simulink model "inverter"  (R2025a)
settings: Solver=FixedStepAuto  StartTime=0.0  StopTime=2  RelTol=1e-3
values from neighbouring files (symbols this model uses):
  Kd = 0    [optimizasyon_baslat.m]
libraries: spsSeriesRLCBranchLib x5, spsDiodeLib x4, spsMosfetLib x4, spsRMSLib x3, spsVoltageMeasurementLib x3, spsControlledVoltageSourceLib x1, spsCurrentMeasurementLib x1, slpidlib x1, eePwmGenerator x1, simulink x1, spsBreakerLib x1, sps_lib x1
settings Model: Creator=TOPALOĞLU  LastModifiedBy=TOPALOĞLU

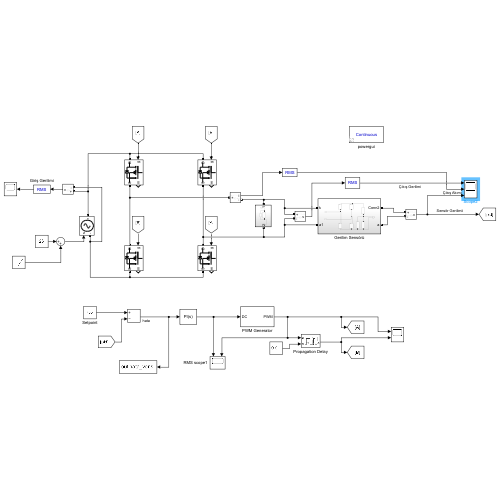
[thumbnail: Simulink's stored preview of the top-level diagram]
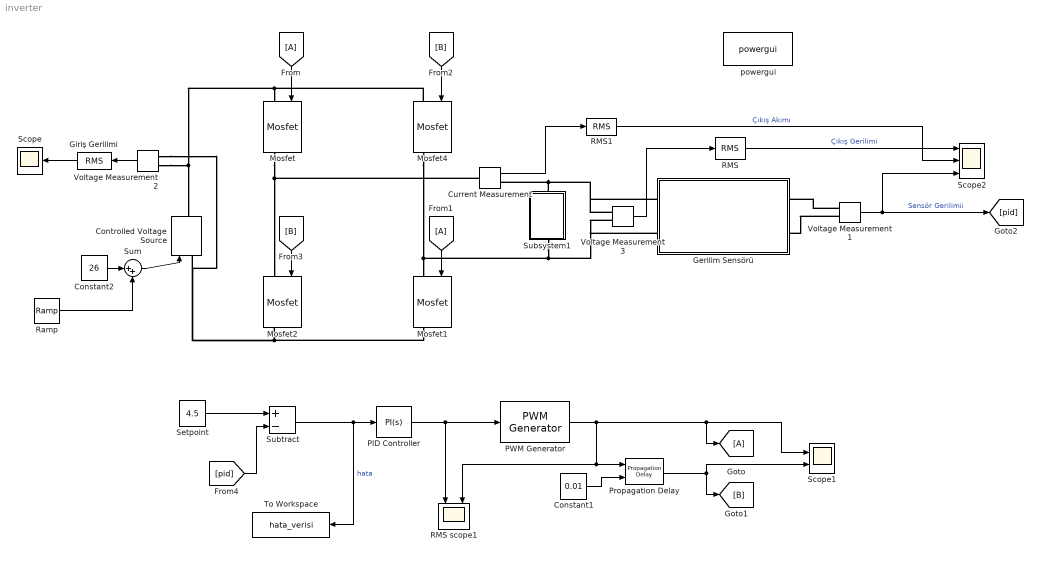
== system inverter ==
  Constant1 : Constant  Value=0.01
  Constant2 : Constant  Value=26
  Controlled Voltage Source : spsControlledVoltageSourceLib/Controlled Voltage Source  Initialize=on  Source_Type=DC  Amplitude=0  Phase=0  Frequency=0  Measurements=None
  Current Measurement : spsCurrentMeasurementLib/Current Measurement  PhasorSimulation=off  OutputType=Complex  PSBequivalent=0
  From : From
  From1 : From
  Gerilim Sensörü : Subsystem
  Giriş Gerilimi : spsRMSLib/RMS  TrueRMS=on  Freq=50  RMSInit=26  Ts=0
  Goto : Goto
  Mosfet{,1..2,4} (4 alike) : spsMosfetLib/Mosfet  Ron=0.1  Lon=0  Rd=0.01  Vfd=0  IC=0  Rs=inf  Cs=0  Measurements=on
  PID Controller : slpidlib/PID Controller  Controller=PI  Form=Parallel  TimeDomain=Continuous-time  UseExternalTs=off  SampleTime=-1  IntegratorMethod=Forward Euler  FilterMethod=Forward Euler  ControllerParametersSource=internal  P=0.059307  I=1.9095  UseKiTs=off  D=Kd  UseExternalDerivativeSource=off  N=100  UseFilter=on  TunerSelectOption=Transfer Function Based (PID Tuner App)  InitialConditionSource=internal  InitialConditionForIntegrator=0  InitialConditionForFilter=0  DifferentiatorICPrevScaledInput=0  ExternalReset=none  TrackingMode=off  Kt=1  LimitOutput=off  SatLimitsSource=internal  UpperSaturationLimit=0.95  LowerSaturationLimit=0  LinearizeAsGain=on  AntiWindupMode=clamping  Kb=1  LimitIntegrator=off  UpperIntegratorSaturationLimit=inf  LowerIntegratorSaturationLimit=-inf  POutMin=[]  POutMax=[]  IOutMin=[]  IOutMax=[]  DOutMin=[]  DOutMax=[]  NOutMin=[]  NOutMax=[]  SumOutMin=[]  SumOutMax=[]  SaturationOutMin=[]  SaturationOutMax=[]  PParamMin=[]  PParamMax=[]  IParamMin=[]  IParamMax=[]  DParamMin=[]  DParamMax=[]  NParamMin=[]  NParamMax=[]  KbParamMin=[]  KbParamMax=[]  KtParamMin=[]  KtParamMax=[]  KbOutMin=[]  KbOutMax=[]  KtOutMin=[]  KtOutMax=[]  IntegratorOutMin=[]  IntegratorOutMax=[]  FilterOutMin=[]  FilterOutMax=[]  SumI1OutMin=[]  SumI1OutMax=[]  SumI2OutMin=[]  SumI2OutMax=[]  SumI3OutMin=[]  SumI3OutMax=[]  SumI4OutMin=[]  SumI4OutMax=[]  SumDOutMin=[]  SumDOutMax=[]  DifferentiatorOutMin=[]  DifferentiatorOutMax=[]  FilterDiffOutCoefMin=[]  FilterDiffOutCoefMax=[]  ReciprocalOutMin=[]  ReciprocalOutMax=[]  SumDenOutMin=[]  SumDenOutMax=[]  SumNumOutMin=[]  SumNumOutMax=[]  DivideOutMin=[]  DivideOutMax=[]  UdiffTsProdOutMin=[]  UdiffTsProdOutMax=[]  NTsProdOutMin=[]  NTsProdOutMax=[]  UintegralTsProdOutMin=[]  UintegralTsProdOutMax=[]  UngainTsProdOutMin=[]  UngainTsProdOutMax=[]  ClampingZeroOutDataTypeStr=Inherit: Inherit via back propagation  ClampingZeroOutMin=[]  ClampingZeroOutMax=[]  FilterDenConstantOutDataTypeStr=Inherit: Inherit via back propagation  FilterDenConstantOutMin=[]  FilterDenConstantOutMax=[]  PCopyOutDataTypeStr=Inherit: Inherit via back propagation  PCopyOutMin=[]  PCopyOutMax=[]  NCopyOutDataTypeStr=Inherit: Inherit via back propagation  NCopyOutMin=[]  NCopyOutMax=[]  IntegratorContinuousStateAttributes=''  IntegratorStateMustResolveToSignalObject=off  IntegratorRTWStateStorageClass=Auto  FilterContinuousStateAttributes=''  FilterStateMustResolveToSignalObject=off  FilterRTWStateStorageClass=Auto  ParallelPVariant=InternalParameters  IdealPVariant=Disabled  IVariant=InternalParameters  DVariant=Disabled  IntegratorVariant=Continuous  SatVariant=Disabled  AWVariant=Passthrough  PCopyVariant=Disabled  TRVariant=Disabled  FdbkBlocksVariant=Forward  IdealPFdbkVariant=Disabled  SatFdbkVariant=Disabled  DerivativeFilterVariant=Disabled  NVariant=Disabled  NCopyVariant=Disabled_SignalSpec  FilterICVariant=Disabled  IntegratorICVariant=InternalICs  ExternalResetVariant=Disabled  TRSumVariant=Passthrough  SumFdbkVariant=Disabled  SumVariant=Sum_PI  TsampFilterVariant=InternalTs  TsampNgainVariant=Passthrough  TsampIntegralVariant=Disabled_SignalSpec  ExternalSaturationOutDataTypeStr=Inherit: Same as second input  DerivativeSourceVariant=Disabled  PreIntVariant=InternalPreInt
  PWM Generator : eePwmGenerator/PWM Generator  CarrCount=Up  Tper=0.02  Tdelay=0  Ts=0
  Propagation Delay : PropagationDelay  RunAtFixedTimeIntervals=on  SampleTime=1e-5
  RMS : spsRMSLib/RMS  TrueRMS=on  Freq=50  RMSInit=12  Ts=0
  RMS scope1 : Scope  NumInputPorts=2
      settings: ActiveDisplayYMinimum=-0.11874999999999997  ActiveDisplayYMaximum=1.0687499999999999
  RMS1 : spsRMSLib/RMS  TrueRMS=on  Freq=50  RMSInit=12  Ts=0
  Ramp : simulink/Sources/Ramp  slope=-2  start=0.3  InitialOutput=0
  Scope : Scope
      settings: ActiveDisplayYMinimum=22.197503315644997  ActiveDisplayYMaximum=26.422499631625165  DataLoggingVariableName=ScopeData2
  Scope1 : Scope  NumInputPorts=2
      settings: SampleTime=5e-5  ActiveDisplayYMinimum=-1.5835891369267512  ActiveDisplayYMaximum=1.8370895793058766
  Scope2 : Scope  NumInputPorts=3
      settings: ActiveDisplayYMinimum=10.998473275040297  ActiveDisplayYMaximum=21.013740524637338  DataLoggingVariableName=ScopeData3
  Setpoint : Constant  Value=4.5
  Subsystem1 : Subsystem
      settings: PortSchema="{\"entries\":[{\"content\":{\"sides\":[{\"content\":{},\"type\":\"ConnectorPlacement.EquallySpacedRectSide\",\"uuid\":\"7486039e-ec59-494d-8c75-0b6bdb988410\"},{\"content\":{\"side\":\"RIGHT\"},\"type\":\"ConnectorPlacement.EquallySpacedRectSide\",\"uuid\":\"15f9885d-5be6-4b9d-bebb-8881537d42c9\"},{\"content\":{\"connectorIds\":[\"LConn1\"],\"side\":\"TOP\"},\"type\":\"ConnectorPlacement.EquallySpacedRectSide\",\"uuid\":\"8cabd63c-7798-48b1-8db3-4643120ccc1c\"},{\"content\":{\"connectorIds\":[\"RConn1\"],\"side\":\"BOTTOM\"},\"type\":\"ConnectorPlacement.EquallySpacedRectSide\",\"uuid\":\"bbf3fb16-ed9b-4739-ac92-1db30e999269\"}]},\"type\":\"ConnectorPlacement.EquallySpacedConnector\",\"uuid\":\"ea19a637-8e2a-4c18-aba2-8529bbc4d327\"}],\"packageUris\":[\"http://schema.mathworks.com/mf0/Connector/R2020b\"],\"version\":\"1.0\"}"
  Subtract : Sum  Inputs=+-
  Sum : Sum  Inputs=|++
  To Workspace : ToWorkspace  VariableName=hata_verisi  SampleTime=-1
      settings: Save2DSignal=2-D array (concatenate along first dimension)
  Voltage Measurement1 : spsVoltageMeasurementLib/Voltage Measurement  PhasorSimulation=off  OutputType=Complex  PSBequivalent=0
  Voltage Measurement2 : spsVoltageMeasurementLib/Voltage Measurement  PhasorSimulation=off  OutputType=Complex  PSBequivalent=0
  Voltage Measurement3 : spsVoltageMeasurementLib/Voltage Measurement  PhasorSimulation=off  OutputType=Complex  PSBequivalent=0
  powergui : sps_lib/powergui  Priority=1  SimulationMode=Continuous  SampleTime=5e-5  frequency=60  Iterations=50  frequencyindice=0  Pbase=100e6  ErrMax=1e-4  UnitsV=kV  UnitsW=MW  buscounter=0  FunctionMessages=off  echomessages=off  EnableUseOfTLC=off  CurrentSourceSwitches=off  DisableSnubberDevices=off  DisableRonSwitches=off  DisableVfSwitches=off  DisplayEquations=off  AutomaticDiscreteSolvers=off  SolverType=Tustin/Backward Euler (TBE)  Interpol=off  ExternalGateDelay=off  methode=off  Ts=100  x0status=blocks  SPID=on  SwTol=0  HookPort=off  NonlinearTolerance=1e-4  nMaxIteration=100  ContinueOnMaxIteration=off  RestoreLinks=warning  ResistiveCurrentMeasurement=off  Frange=[0:2:500]  Ylog=off  Xlog=on  ShowGrid=off  save=off  variable=ZData  structure=0  ZoomFFT=off  StartTime=0.0  cycles=1  DisplayStyle=1  fundamental=60  FreqAxis=off  MaxFrequency=1000  frequencyindicesteady=1  RmsSteady=1  display=off
  wires:
  [B] -> Mosfet4/1
  From1/1 -> Mosfet1/1
  Constant1/1 -> Propagation Delay/2
  Setpoint/1 -> Subtract/1
  Subtract/1 -> To Workspace/1, PID Controller/1  "hata"
  [B] -> Mosfet2/1
  PWM Generator/1 -> Propagation Delay/1, RMS scope1/2, Goto/1, Scope1/1
  From/1 -> Mosfet/1
  Propagation Delay/1 -> Scope1/2, [B]
  Constant2/1 -> Sum/1
  Ramp/1 -> Sum/2
  Sum/1 -> Controlled Voltage Source/1
  Giriş Gerilimi/1 -> Scope/1
  Voltage Measurement2/1 -> Giriş Gerilimi/1
  Voltage Measurement3/1 -> RMS/1
  RMS/1 -> Scope2/1  "Çıkış Gerilimi"
  Voltage Measurement1/1 -> [pid], Scope2/3  "Sensör Gerilimii"
  PID Controller/1 -> PWM Generator/1, RMS scope1/1
  Current Measurement/1 -> RMS1/1
  RMS1/1 -> Scope2/2  "Çıkış Akımı"
  [pid] -> Subtract/2
  connections:
  Mosfet4/LConn1 -- Voltage Measurement2/LConn1 -- Controlled Voltage Source/RConn1 -- Mosfet/LConn1
  Mosfet1/RConn1 -- Voltage Measurement2/LConn2 -- Controlled Voltage Source/LConn1 -- Mosfet2/RConn1
  Mosfet/RConn1 -- Current Measurement/LConn1 -- Mosfet2/LConn1
  Mosfet4/RConn1 -- Voltage Measurement3/LConn2 -- Gerilim Sensörü/LConn2 -- Subsystem1/RConn1 -- Mosfet1/LConn1
  Subsystem1/LConn1 -- Gerilim Sensörü/LConn1 -- Voltage Measurement3/LConn1 -- Current Measurement/RConn1
  Voltage Measurement1/LConn1 -- Gerilim Sensörü/RConn1
  Voltage Measurement1/LConn2 -- Gerilim Sensörü/RConn2

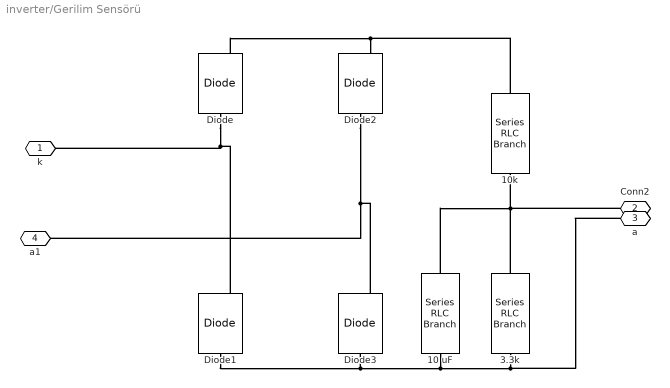
== system inverter/Gerilim Sensörü ==
  10 uF : spsSeriesRLCBranchLib/Series RLC Branch  LConnTagsString=__new0  RConnTagsString=__new0  BranchType=C  Resistance=1  Inductance=1e-3  SetiL0=off  InitialCurrent=0  Capacitance=10e-6  Setx0=off  InitialVoltage=0  Measurements=None
  10k : spsSeriesRLCBranchLib/Series RLC Branch  LConnTagsString=__new0  RConnTagsString=__new0  BranchType=R  Resistance=10000  Inductance=1e-3  SetiL0=off  InitialCurrent=0  Capacitance=10e-6  Setx0=off  InitialVoltage=0  Measurements=None
  3.3k : spsSeriesRLCBranchLib/Series RLC Branch  LConnTagsString=__new0  RConnTagsString=__new0  BranchType=R  Resistance=3300  Inductance=1e-3  SetiL0=off  InitialCurrent=0  Capacitance=10e-6  Setx0=off  InitialVoltage=0  Measurements=None
  Diode{,1..3} (4 alike) : spsDiodeLib/Diode  Ron=0.001  Lon=0  Vf=0.8  IC=0  UseSnubber=0  Rs=500  Cs=250e-9  Measurements=on
  k : PMIOPort  Side=Left
  Conn2 : PMIOPort  Port=2  Side=Right
  a : PMIOPort  Port=3  Side=Right
  a1 : PMIOPort  Port=4  Side=Left
  connections:
  Diode1/LConn1 -- 10 uF/RConn1 -- a/RConn1 -- 3.3k/RConn1 -- Diode3/LConn1
  Diode/LConn1 -- k/RConn1 -- Diode1/RConn1
  Diode3/RConn1 -- a1/RConn1 -- Diode2/LConn1
  3.3k/LConn1 -- Conn2/RConn1 -- 10 uF/LConn1 -- 10k/RConn1
  Diode/RConn1 -- 10k/LConn1 -- Diode2/RConn1

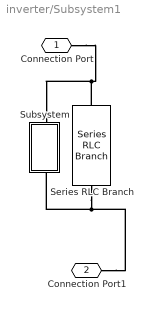
== system inverter/Subsystem1 ==
  Series RLC Branch : spsSeriesRLCBranchLib/Series RLC Branch  LConnTagsString=__new0  RConnTagsString=__new0  BranchType=R  Resistance=2.2  Inductance=1e-3  SetiL0=off  InitialCurrent=0  Capacitance=1e-6  Setx0=off  InitialVoltage=0  Measurements=None
  Subsystem : Subsystem
      settings: PortSchema="{\"entries\":[{\"content\":{\"sides\":[{\"content\":{},\"type\":\"ConnectorPlacement.EquallySpacedRectSide\",\"uuid\":\"0b54102a-f52c-4efd-9575-bdc9cbb2ad90\"},{\"content\":{\"side\":\"RIGHT\"},\"type\":\"ConnectorPlacement.EquallySpacedRectSide\",\"uuid\":\"1646f846-0a53-43cd-a3d0-f9f8e311844b\"},{\"content\":{\"connectorIds\":[\"LConn1\"],\"side\":\"TOP\"},\"type\":\"ConnectorPlacement.EquallySpacedRectSide\",\"uuid\":\"7403264c-1878-4f94-847c-0c2ca458d800\"},{\"content\":{\"connectorIds\":[\"RConn1\"],\"side\":\"BOTTOM\"},\"type\":\"ConnectorPlacement.EquallySpacedRectSide\",\"uuid\":\"8c447138-c617-4ed8-bc80-6919fea9d7a8\"}]},\"type\":\"ConnectorPlacement.EquallySpacedConnector\",\"uuid\":\"d5635a6b-c386-4653-92b0-90d86cdb9e8b\"}],\"packageUris\":[\"http://schema.mathworks.com/mf0/Connector/R2020b\"],\"version\":\"1.0\"}"
  Connection Port : PMIOPort  Side=Left
  Connection Port1 : PMIOPort  Port=2  Side=Right
  connections:
  Series RLC Branch/RConn1 -- Connection Port1/RConn1 -- Subsystem/RConn1
  Series RLC Branch/LConn1 -- Connection Port/RConn1 -- Subsystem/LConn1

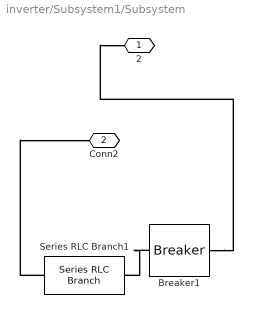
== system inverter/Subsystem1/Subsystem ==
  Breaker1 : spsBreakerLib/Breaker  InitialState=0  SwitchingTimes=[0.7 1.5]  External=off  BreakerResistance=0.01  SnubberResistance=1e6  SnubberCapacitance=inf  Measurements=None  MoreParameters=on  NoBreakLoop=off
  Series RLC Branch1 : spsSeriesRLCBranchLib/Series RLC Branch  LConnTagsString=__new0  RConnTagsString=__new0  BranchType=R  Resistance=2.2  Inductance=1e-3  SetiL0=off  InitialCurrent=0  Capacitance=1e-6  Setx0=off  InitialVoltage=0  Measurements=None
  2 : PMIOPort  Side=Left
  Conn2 : PMIOPort  Port=2  Side=Right
  connections:
  Breaker1/LConn1 -- Series RLC Branch1/LConn1
  Breaker1/RConn1 -- 2/RConn1
  Series RLC Branch1/RConn1 -- Conn2/RConn1
